simulink model "Full_model"  (R2019b)
settings: Solver=VariableStepAuto  StartTime=0.0  StopTime=150  RelTol=1e-3
model workspace: external: MATLAB File C:\Users\Techboard IITG\Downloads\Simscape4\Full_assem_DataFile.m (data not in the file)
undefined symbols (not defined in the file): _Default_sldprt, apx, ch_app, ch_cyc, cpz, L1, L2, L2rz, L2xf, L2yf, L2zf, l_app, max_avel, max_tvel, smiData, stand, TH1_ec_i, TH1_f, TH1_i, TH1_i_r, TH1_ri, TH2_ec_i, TH2_f, TH2_i, TH2_i_r, TH2_ri, TH3_f, TH3_i, TH3_ri, TH4_f, TH4_i, TH4_ri, time_ch_app, time_if, time_plug, time_ri, time_zchapp_down, time_zchapp_up, X, xp_dist, xp_vel, xpf_i, Y, yp_dist, yp_vel, ypf_i, Z, z_chapp, Z_i, zp_dist, zp_vel, zpf_i
libraries: simulink x68, fl_lib x36, sm_lib x22, nesl_utility x21, ee_lib x12
(part 3 of 3)

== system Full_model/TRAJECTORY_PLANNING/Z_Interpolation/IF_INTER5 ==
  note: set waypt. theta1
  Z_i : Inport
  Z : Inport  Port=2
  MATLAB Function14 : MATLAB Function  TreatAsAtomicUnit=on
  Saturation Dynamic12 : simulink/Discontinuities/Saturation Dynamic  OutMin=[]  OutMax=[]  OutDataTypeStr=Inherit: Same as second input  OutDataType=fixdt(1, 16)  OutScaling=2^-10  DoSatur=off
  Switch16 : Switch  Criteria=u2 > Threshold
  r_neg12 : simulink/Sources/Ramp  slope=-max_tvel  start=(time_ri+time_ch_app-time_zchapp_down)  InitialOutput=0
  r_pos12 : simulink/Sources/Ramp  slope=max_tvel  start=(time_ri+time_ch_app-time_zchapp_down)  InitialOutput=0
  y : Outport
  wires:
  Z_i/1 -> MATLAB Function14/1(Z_i)
  Z/1 -> MATLAB Function14/2(Z)
  r_pos12/1 -> Switch16/1
  Saturation Dynamic12/1 -> y/1
  r_neg12/1 -> Switch16/3
  Switch16/1 -> Saturation Dynamic12/2
  MATLAB Function14/1(u) -> Saturation Dynamic12/1
  MATLAB Function14/2(y) -> Switch16/2
  MATLAB Function14/3(l) -> Saturation Dynamic12/3

== system Full_model/TRAJECTORY_PLANNING/Z_Interpolation/IF_INTER6 ==
  note: set waypt. theta1
  Z_i : Inport
  Z : Inport  Port=2
  MATLAB Function14 : MATLAB Function  TreatAsAtomicUnit=on
  Saturation Dynamic12 : simulink/Discontinuities/Saturation Dynamic  OutMin=[]  OutMax=[]  OutDataTypeStr=Inherit: Same as second input  OutDataType=fixdt(1, 16)  OutScaling=2^-10  DoSatur=off
  Switch16 : Switch  Criteria=u2 > Threshold
  r_neg12 : simulink/Sources/Ramp  slope=-max_avel  start=time_ri  InitialOutput=0
  r_pos12 : simulink/Sources/Ramp  slope=max_tvel  start=time_ri  InitialOutput=0
  y : Outport
  wires:
  Z_i/1 -> MATLAB Function14/1(Z_i)
  Z/1 -> MATLAB Function14/2(Z)
  r_pos12/1 -> Switch16/1
  Saturation Dynamic12/1 -> y/1
  r_neg12/1 -> Switch16/3
  Switch16/1 -> Saturation Dynamic12/2
  MATLAB Function14/1(u) -> Saturation Dynamic12/1
  MATLAB Function14/2(y) -> Switch16/2
  MATLAB Function14/3(l) -> Saturation Dynamic12/3

== system Full_model/TRAJECTORY_PLANNING/Z_Interpolation/IF_INTER7 ==
  note: set waypt. theta1
  Z_i : Inport
  Z : Inport  Port=2
  MATLAB Function14 : MATLAB Function  TreatAsAtomicUnit=on
  Saturation Dynamic12 : simulink/Discontinuities/Saturation Dynamic  OutMin=[]  OutMax=[]  OutDataTypeStr=Inherit: Same as second input  OutDataType=fixdt(1, 16)  OutScaling=2^-10  DoSatur=off
  Switch16 : Switch  Criteria=u2 > Threshold
  r_neg12 : simulink/Sources/Ramp  slope=-max_tvel  start=(time_ri+time_ch_app+time_if+(2*time_plug)+ch_cyc+5)  InitialOutput=0
  r_pos12 : simulink/Sources/Ramp  slope=max_tvel  start=(time_ri+time_ch_app+time_if+(2*time_plug)+ch_cyc+5)  InitialOutput=0
  y : Outport
  wires:
  Z_i/1 -> MATLAB Function14/1(Z_i)
  Z/1 -> MATLAB Function14/2(Z)
  r_pos12/1 -> Switch16/1
  Saturation Dynamic12/1 -> y/1
  r_neg12/1 -> Switch16/3
  Switch16/1 -> Saturation Dynamic12/2
  MATLAB Function14/1(u) -> Saturation Dynamic12/1
  MATLAB Function14/2(y) -> Switch16/2
  MATLAB Function14/3(l) -> Saturation Dynamic12/3

== matlab function Full_model/FORWARD KINEMATICS ==
  data: X output; TH1 input; TH2 input; TH3 input; TH4 input; Z_val input; Y output; Z output
function [X,Y,Z] = FK_BLOCK(TH1,TH2,TH3,TH4,Z_val)

L1 = 0.54;
L2 = 0.475;

yos = 0.128;
p_dist = 0.2285-0.145;
dfp = 0;

h = p_dist/cos(TH4);
b = p_dist/cot(TH4); % y for just off of surface of port

TH3_new = TH3 + (TH1+TH2);

% change 0.128 to 0.135
% for stopping x cm away from port change 0.128 to (0.128+x)
% plugging in distance required 3.3cm + x

vn_sclr = yos+dfp+b; % scaling factor for unit vector vn
  offx = -(vn_sclr)*(cos(TH4)*cos(TH3_new));
  offy = -(vn_sclr)*(cos(TH4)*sin(TH3_new));
  offz = -(vn_sclr)*(sin(TH4)) + 0.145 + h;

X = L1*cos(TH1) + L2*cos(TH1+TH2) - offx;
Y = L1*sin(TH1) + L2*sin(TH1+TH2) - offy;
Z = Z_val - offz;

end

== matlab function Full_model/TRAJECTORY_PLANNING/CHAPP_INTER1/MATLAB Function12 ==
  data: u output; TH_i input; y output; TH input; l output
function [u,y,l] = ramp_sel(TH_i,TH)
if TH_i<TH
    y = 1;
    u = TH-TH_i;
    l = 0;
else
    y = -1;
    u = 0;
    l = TH-TH_i;
end

== matlab function Full_model/TRAJECTORY_PLANNING/CHAPP_INTER2/MATLAB Function13 ==
  data: TH input; TH_i input; u output; y output; l output
function [u,y,l] = ramp_sel(TH,TH_i)
if TH_i<TH
    y = 1;
    u = TH-TH_i;
    l = 0;
else
    y = -1;
    u = 0;
    l = TH-TH_i;
end

== matlab function Full_model/TRAJECTORY_PLANNING/IF_INTER1/MATLAB Function14 ==
  data: u output; TH_i input; y output; TH input; l output
function [u,y,l] = ramp_sel(TH_i,TH)
if TH_i<TH
    y = 1;
    u = TH-TH_i;
    l = 0;
else
    y = -1;
    u = 0;
    l = TH-TH_i;
end

== matlab function Full_model/TRAJECTORY_PLANNING/IF_INTER2/MATLAB Function15 ==
  data: TH input; u output; TH_i input; y output; l output
function [u,y,l] = ramp_sel(TH,TH_i)
if TH_i<TH
    y = 1;
    u = TH-TH_i;
    l = 0;
else
    y = -1;
    u = 0;
    l = TH-TH_i;
end

== matlab function Full_model/TRAJECTORY_PLANNING/IF_INTER3/MATLAB Function14 ==
  data: u output; TH_i input; y output; TH input; l output
function [u,y,l] = ramp_sel(TH_i,TH)
if TH_i<TH
    y = 1;
    u = TH-TH_i;
    l = 0;
else
    y = -1;
    u = 0;
    l = TH-TH_i;
end

== matlab function Full_model/TRAJECTORY_PLANNING/IF_INTER4/MATLAB Function15 ==
  data: TH input; u output; TH_i input; y output; l output
function [u,y,l] = ramp_sel(TH,TH_i)
if TH_i<TH
    y = 1;
    u = TH-TH_i;
    l = 0;
else
    y = -1;
    u = 0;
    l = TH-TH_i;
end

== matlab function Full_model/TRAJECTORY_PLANNING/Subsystem/MATLAB Function10 ==
  data: u output; TH_i input; y output; TH input; l output
function [u,y,l] = ramp_sel(TH_i,TH)
if TH_i<TH
    y = 1;
    u = TH;
    l = TH_i;
else
    y = -1;
    u = TH_i;
    l = TH;
end

== matlab function Full_model/TRAJECTORY_PLANNING/Subsystem1/MATLAB Function11 ==
  data: TH input; u output; TH_i input; y output; l output
function [u,y,l] = ramp_sel(TH,TH_i)
if TH_i<TH
    y = 1;
    u = TH;
    l = TH_i;
else
    y = -1;
    u = TH_i;
    l = TH;
end

== matlab function Full_model/TRAJECTORY_PLANNING/TH3_Interpolation/IF_INTER1/MATLAB Function14 ==
  data: u output; TH_i input; y output; TH input; l output
function [u,y,l] = ramp_sel(TH_i,TH)
if TH_i<TH
    y = 1;
    u = TH-TH_i;
    l = 0;
else
    y = -1;
    u = 0;
    l = TH-TH_i;
end

== matlab function Full_model/TRAJECTORY_PLANNING/TH3_Interpolation/IF_INTER2/MATLAB Function14 ==
  data: u output; TH_i input; y output; TH input; l output
function [u,y,l] = ramp_sel(TH_i,TH)
if TH_i<TH
    y = 1;
    u = TH-TH_i;
    l = 0;
else
    y = -1;
    u = 0;
    l = TH-TH_i;
end

== matlab function Full_model/TRAJECTORY_PLANNING/TH3_Interpolation/IF_INTER3/MATLAB Function14 ==
  data: u output; TH_i input; y output; TH input; l output
function [u,y,l] = ramp_sel(TH_i,TH)
if TH_i<TH
    y = 1;
    u = TH;
    l = TH_i;
else
    y = -1;
    u = TH_i;
    l = TH;
end

== matlab function Full_model/TRAJECTORY_PLANNING/TH4_Interpolation/IF_INTER1/MATLAB Function14 ==
  data: u output; TH_i input; y output; TH input; l output
function [u,y,l] = ramp_sel(TH_i,TH)
if TH_i<TH
    y = 1;
    u = TH-TH_i;
    l = 0;
else
    y = -1;
    u = 0;
    l = TH-TH_i;
end

== matlab function Full_model/TRAJECTORY_PLANNING/TH4_Interpolation/IF_INTER2/MATLAB Function14 ==
  data: u output; TH_i input; y output; TH input; l output
function [u,y,l] = ramp_sel(TH_i,TH)
if TH_i<TH
    y = 1;
    u = TH-TH_i;
    l = 0;
else
    y = -1;
    u = 0;
    l = TH-TH_i;
end

== matlab function Full_model/TRAJECTORY_PLANNING/TH4_Interpolation/IF_INTER5/MATLAB Function14 ==
  data: u output; TH_i input; y output; TH input; l output
function [u,y,l] = ramp_sel(TH_i,TH)
if TH_i<TH
    y = 1;
    u = TH;
    l = TH_i;
else
    y = -1;
    u = TH_i;
    l = TH;
end

== matlab function Full_model/TRAJECTORY_PLANNING/TS_JA_Interpolation/IK_BLOCK1/MATLAB Function ==
  data: TH1_1 input; TH1 output; TH1_2 input; TH2_2 input; TH2_1 input; TH2 output; l_app input
function [TH1,TH2] = anyapp(TH1_1,TH1_2,TH2_2,TH2_1,l_app)

if l_app == -1
    if TH2_1<0
        TH1 = TH1_2;
        TH2 = TH2_2;
    else
        TH1 = TH1_1;
        TH2 = TH2_1;
    end
else
    if TH2_1>0
        TH1 = TH1_2;
        TH2 = TH2_2;
    else
        TH1 = TH1_1;
        TH2 = TH2_1;
    end
end

== matlab function Full_model/TRAJECTORY_PLANNING/TS_JA_Interpolation/IK_BLOCK1/TH1_1 ==
  data: L_1 input; out1 output; L_2 input; XE input; YE input
function out1 = TH1_1(L_1,L_2,XE,YE)
%#codegen

%    This function was generated by the Symbolic Math Toolbox version 9.2.
%    29-Jan-2023 18:29:05

t2 = L_1.^2;
t3 = L_2.^2;
t4 = XE.^2;
t5 = YE.^2;
t6 = L_1.*L_2.*2.0;
t7 = -t2;
t8 = -t3;
t9 = -t4;
t10 = -t5;
t11 = t4+t5+t6+t7+t8;
t12 = t2+t3+t6+t9+t10;
t13 = 1.0./t11;
t14 = t11.*t12;
t15 = sqrt(t14);
out1 = atan((L_1.*YE.*2.0+t4.*t13.*t15+t5.*t13.*t15+t6.*t13.*t15+t7.*t13.*t15+t8.*t13.*t15)./(t2+t4+t5+t8+L_1.*XE.*2.0)).*2.0;

== matlab function Full_model/TRAJECTORY_PLANNING/TS_JA_Interpolation/IK_BLOCK1/TH1_2 ==
  data: L_1 input; out1 output; L_2 input; XE input; YE input
function out1 = TH1_2(L_1,L_2,XE,YE)
%#codegen

%    This function was generated by the Symbolic Math Toolbox version 9.2.
%    29-Jan-2023 18:29:05

t2 = L_1.^2;
t3 = L_2.^2;
t4 = XE.^2;
t5 = YE.^2;
t6 = L_1.*L_2.*2.0;
t7 = -t2;
t8 = -t3;
t9 = -t4;
t10 = -t5;
t11 = t4+t5+t6+t7+t8;
t12 = t2+t3+t6+t9+t10;
t13 = 1.0./t11;
t14 = t11.*t12;
t15 = sqrt(t14);
out1 = atan((L_1.*YE.*2.0+t2.*t13.*t15+t3.*t13.*t15+t9.*t13.*t15+t10.*t13.*t15-L_1.*L_2.*t13.*t15.*2.0)./(t2+t4+t5+t8+L_1.*XE.*2.0)).*2.0;

== matlab function Full_model/TRAJECTORY_PLANNING/TS_JA_Interpolation/IK_BLOCK1/TH2_1 ==
  data: L_1 input; out1 output; L_2 input; XE input; YE input
function out1 = TH2_1(L_1,L_2,XE,YE)
%#codegen

%    This function was generated by the Symbolic Math Toolbox version 9.2.
%    29-Jan-2023 18:29:05

t2 = L_1.^2;
t3 = L_2.^2;
t4 = XE.^2;
t5 = YE.^2;
t6 = L_1.*L_2.*2.0;
t7 = -t2;
t8 = -t3;
t9 = t4+t5+t6+t7+t8;
out1 = atan(sqrt(t9.*(t2+t3-t4-t5+t6))./t9).*-2.0;

== matlab function Full_model/TRAJECTORY_PLANNING/TS_JA_Interpolation/IK_BLOCK1/TH2_2 ==
  data: L_1 input; out1 output; L_2 input; XE input; YE input
function out1 = TH2_2(L_1,L_2,XE,YE)
%#codegen

%    This function was generated by the Symbolic Math Toolbox version 9.2.
%    29-Jan-2023 18:29:06

t2 = L_1.^2;
t3 = L_2.^2;
t4 = XE.^2;
t5 = YE.^2;
t6 = L_1.*L_2.*2.0;
t7 = -t2;
t8 = -t3;
t9 = t4+t5+t6+t7+t8;
out1 = atan(sqrt(t9.*(t2+t3-t4-t5+t6))./t9).*2.0;

== matlab function Full_model/TRAJECTORY_PLANNING/Z_Interpolation/CHAPP_INTER3/MATLAB Function12 ==
  data: u output; Z_i input; y output; Z input; l output
function [u,y,l] = ramp_sel(Z_i,Z)
if Z_i<Z
    y = 1;
    u = Z;
    l = Z_i;
else
    y = -1;
    u = Z_i;
    l = Z;
end

== matlab function Full_model/TRAJECTORY_PLANNING/Z_Interpolation/CHAPP_INTER4/MATLAB Function12 ==
  data: u output; Z_i input; y output; zpf input; l output
function [u,y,l] = ramp_sel(Z_i,zpf)
if Z_i<zpf
    y = 1;
    u = zpf-Z_i;
    l = 0;
else
    y = -1;
    u = 0;
    l = zpf-Z_i;
end

== matlab function Full_model/TRAJECTORY_PLANNING/Z_Interpolation/IF_INTER5/MATLAB Function14 ==
  data: u output; Z_i input; y output; Z input; l output
function [u,y,l] = ramp_sel(Z_i,Z)
if Z_i<Z
    y = 1;
    u = Z-Z_i;
    l = 0;
else
    y = -1;
    u = 0;
    l = Z-Z_i;
end

== matlab function Full_model/TRAJECTORY_PLANNING/Z_Interpolation/IF_INTER6/MATLAB Function14 ==
  data: u output; Z_i input; y output; Z input; l output
function [u,y,l] = ramp_sel(Z_i,Z)
if Z_i<Z
    y = 1;
    u = Z-Z_i;
    l = 0;
else
    y = -1;
    u = 0;
    l = Z-Z_i;
end

== matlab function Full_model/TRAJECTORY_PLANNING/Z_Interpolation/IF_INTER7/MATLAB Function14 ==
  data: u output; Z_i input; y output; Z input; l output
function [u,y,l] = ramp_sel(Z_i,Z)
if Z_i<Z
    y = 1;
    u = Z-Z_i;
    l = 0;
else
    y = -1;
    u = 0;
    l = Z-Z_i;
end
